simulink model "submited-as-classwork--week_2_simulink_model"  (R2023b)
settings: Solver=VariableStepAuto  StartTime=0.0  StopTime=10  RelTol=1e-3
settings Model: Creator=Aksel Cavak  LastModifiedBy=Aksel Cavak

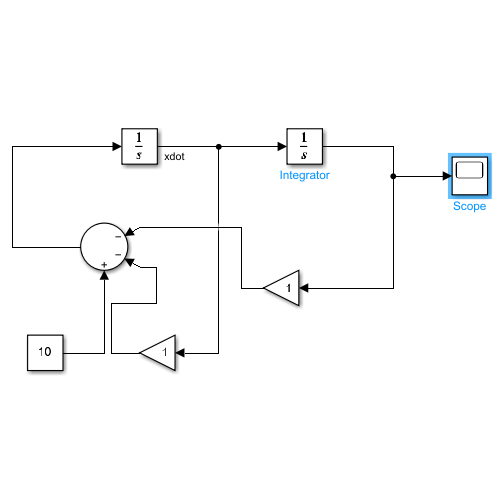
[thumbnail: Simulink's stored preview of the top-level diagram]
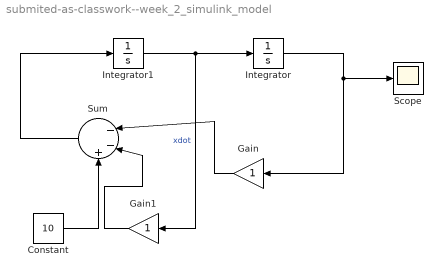
== system submited-as-classwork--week_2_simulink_model ==
  Constant : Constant  Value=10
  Gain : Gain
  Gain1 : Gain
  Integrator : Integrator  InitialCondition=6
  Integrator1 : Integrator  InitialCondition=3
  Scope : Scope
  Sum : Sum  Inputs=|--+
  wires:
  Integrator/1 -> Gain/1, Scope/1
  Integrator1/1 -> Gain1/1, Integrator/1  "xdot"
  Gain1/1 -> Sum/2
  Gain/1 -> Sum/1
  Constant/1 -> Sum/3
  Sum/1 -> Integrator1/1
